simulink library "UserContent_lib"  (Simulink 7.2)
settings: Solver=ode45  SolverMode=SingleTasking  StartTime=0.0  StopTime=10.0  RelTol=1e-3
undefined symbols (not defined in the file or in its folder): bias, Timestep, WindDir, WindSpd
libraries: aeroutilslib x4, First_Order_Filter_lib x4, simulink x1, timer_lib x1
settings Model: Creator=Austin Murch  LastModifiedBy=la1032aw  ExtModeAutoUpdateStatusClock=off

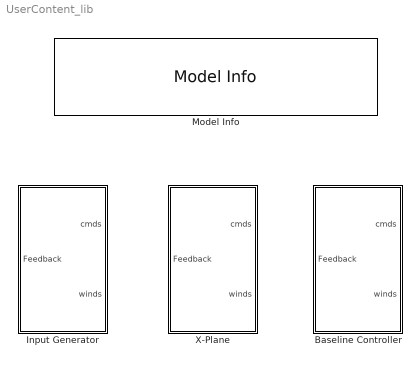
== system UserContent_lib ==
  Baseline Controller : Subsystem
  Input Generator : Subsystem
  Model Info : simulink/Model-Wide Utilities/Model Info  SystemSampleTime=-1  InitialBlockCM=None  BlockCM=None  Frame=on  DisplayStringWithTags=|  HorizontalTextAlignment=Center  LeftAlignmentValue=0.5  SourceBlockDiagram=UserContent_lib  TagMaxNumber=20
      | - gtm_design Input Library -
      | 
      | Model Version: %<ModelVersion>
      | Last modifed by %<LastModifiedBy> on %<LastModificationDate>
  X-Plane : Subsystem

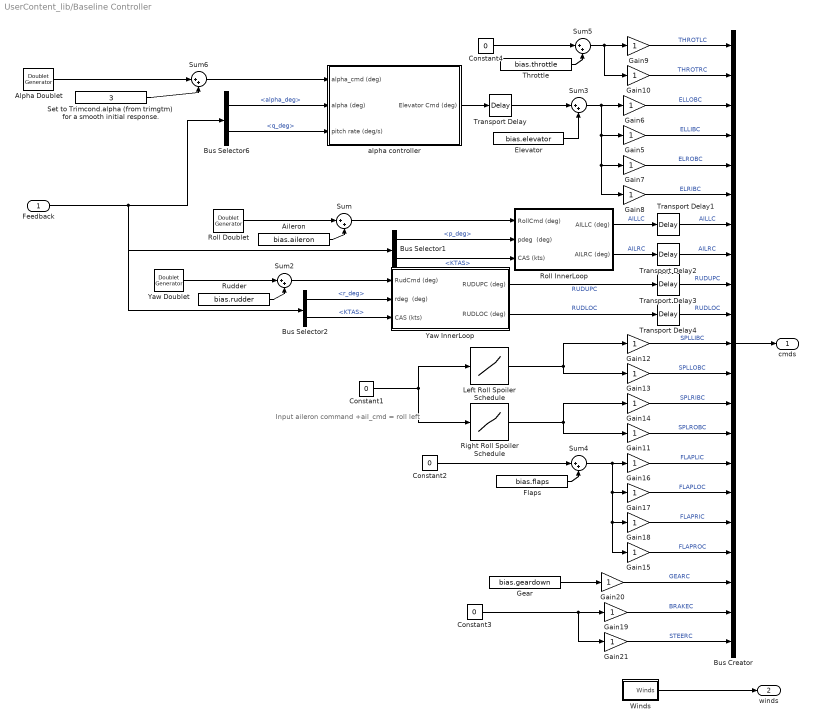
== system UserContent_lib/Baseline Controller ==
  note: Input aileron command
      | +ail_cmd = roll left
  Feedback : Inport  OutDataType=sfix(16)  OutScaling=2^0
  Aileron : Constant  Value=bias.aileron  OutDataType=sfix(16)  OutScaling=2^0
  Alpha Doublet : aeroutilslib/Doublet Generator  SystemSampleTime=-1  timeon=2  pulsewidth=2  amplitude=1
  Bus Creator : BusCreator  Inputs=21
  Bus Selector1 : BusSelector  OutputSignals=MAG3.p_deg,AirData.KTAS
  Bus Selector2 : BusSelector  OutputSignals=MAG3.r_deg,AirData.KTAS
  Bus Selector6 : BusSelector  OutputSignals=AirData.alpha_deg,MAG3.q_deg
  Constant{1..4} (4 alike) : Constant  Value=0  OutDataType=sfix(16)  OutScaling=2^0
  Elevator : Constant  Value=bias.elevator  OutDataType=sfix(16)  OutScaling=2^0
  Flaps : Constant  Value=bias.flaps  OutDataType=sfix(16)  OutScaling=2^0
  Gain{5..21} (17 alike) : Gain  ParameterDataType=sfix(16)  ParameterScaling=2^0  OutDataType=sfix(16)  OutScaling=2^0  SaturateOnIntegerOverflow=on  OutDataTypeStr=Inherit: Same as input  ParamDataTypeStr=Inherit: Same as input
  Gear : Constant  Value=bias.geardown  OutDataType=sfix(16)  OutScaling=2^0
  Left Roll Spoiler Schedule : Lookup  InputValues="[-20\t-11.76\t-2.36\t0\t2.36\t11.76\t20\t]"  Table=[0 0 0 0 0 9 45]  LookUpMeth=Interpolation-Use End Values  OutDataType=sfix(16)  OutScaling=2^0
  Right Roll Spoiler Schedule : Lookup  InputValues="[-20\t-11.76\t-2.36\t0\t2.36\t11.76\t20\t]"  Table=[45 9 0 0 0 0 0]  LookUpMeth=Interpolation-Use End Values  OutDataType=sfix(16)  OutScaling=2^0
  Roll Doublet : aeroutilslib/Doublet Generator  SystemSampleTime=-1  timeon=8  pulsewidth=2  amplitude=1
  Roll InnerLoop : Subsystem
  Rudder : Constant  Value=bias.rudder  OutDataType=sfix(16)  OutScaling=2^0
  Set to Trimcond.alpha (from trimgtm)  for a smooth initial response. : Constant  Value=3  OutDataType=sfix(16)  OutScaling=2^0
  Sum{,2..6} (6 alike) : Sum  Inputs=|++  OutDataType=sfix(16)  OutScaling=2^0
  Throttle : Constant  Value=bias.throttle  OutDataType=sfix(16)  OutScaling=2^0
  Transport Delay{,1..4} (5 alike) : TransportDelay  DelayTime=20e-3
  Winds : Subsystem
  Yaw Doublet : aeroutilslib/Doublet Generator  SystemSampleTime=-1  timeon=12  pulsewidth=2  amplitude=1
  Yaw InnerLoop : Subsystem
  alpha controller : Subsystem
  cmds : Outport  OutDataType=sfix(16)  OutScaling=2^0
  winds : Outport  Port=2  OutDataType=sfix(16)  OutScaling=2^0
  wires:
  Yaw Doublet/1 -> Sum2/1
  Roll Doublet/1 -> Sum/1
  Bus Selector2/2 -> Yaw InnerLoop/3(CAS (kts))  "<KTAS>"
  Bus Selector2/1 -> Yaw InnerLoop/2(rdeg  (deg))  "<r_deg>"
  Bus Selector1/2 -> Roll InnerLoop/3(CAS (kts))  "<KTAS>"
  Bus Selector1/1 -> Roll InnerLoop/2(pdeg  (deg))  "<p_deg>"
  Sum2/1 -> Yaw InnerLoop/1(RudCmd (deg))
  Rudder/1 -> Sum2/2
  Sum/1 -> Roll InnerLoop/1(RollCmd (deg))
  alpha controller/1(Elevator Cmd (deg)) -> Transport Delay/1
  Bus Selector6/1 -> alpha controller/2(alpha (deg))  "<alpha_deg>"
  Sum6/1 -> alpha controller/1(alpha_cmd (deg))
  Alpha Doublet/1 -> Sum6/1
  Set to Trimcond.alpha (from trimgtm)  for a smooth initial response./1 -> Sum6/2
  Gain12/1 -> Bus Creator/11  "SPLLIBC"
  Gain13/1 -> Bus Creator/12  "SPLLOBC"
  Gain14/1 -> Bus Creator/13  "SPLRIBC"
  Gain11/1 -> Bus Creator/14  "SPLROBC"
  Gain16/1 -> Bus Creator/15  "FLAPLIC"
  Gain17/1 -> Bus Creator/16  "FLAPLOC"
  Gain18/1 -> Bus Creator/17  "FLAPRIC"
  Gain15/1 -> Bus Creator/18  "FLAPROC"
  Gain9/1 -> Bus Creator/1  "THROTLC"
  Gain10/1 -> Bus Creator/2  "THROTRC"
  Gain5/1 -> Bus Creator/4  "ELLIBC"
  Gain6/1 -> Bus Creator/3  "ELLOBC"
  Gain7/1 -> Bus Creator/5  "ELROBC"
  Gain8/1 -> Bus Creator/6  "ELRIBC"
  Roll InnerLoop/1(AILLC (deg)) -> Transport Delay1/1  "AILLC"
  Roll InnerLoop/2(AILRC (deg)) -> Transport Delay2/1  "AILRC"
  Yaw InnerLoop/1(RUDUPC (deg)) -> Transport Delay3/1  "RUDUPC"
  Yaw InnerLoop/2(RUDLOC (deg)) -> Transport Delay4/1  "RUDLOC"
  Throttle/1 -> Sum5/2
  Constant4/1 -> Sum5/1
  Sum5/1 -> Gain10/1, Gain9/1
  Sum3/1 -> Gain6/1, Gain5/1, Gain7/1, Gain8/1
  Aileron/1 -> Sum/2
  Elevator/1 -> Sum3/2
  Flaps/1 -> Sum4/2
  Constant2/1 -> Sum4/1
  Sum4/1 -> Gain16/1, Gain17/1, Gain18/1, Gain15/1
  Gain19/1 -> Bus Creator/20  "BRAKEC"
  Gear/1 -> Gain20/1
  Constant3/1 -> Gain19/1, Gain21/1
  Bus Creator/1 -> cmds/1
  Feedback/1 -> Bus Selector6/1, Bus Selector2/1, Bus Selector1/1
  Gain20/1 -> Bus Creator/19  "GEARC"
  Gain21/1 -> Bus Creator/21  "STEERC"
  Bus Selector6/2 -> alpha controller/3(pitch rate (deg/s))  "<q_deg>"
  Left Roll Spoiler Schedule/1 -> Gain12/1, Gain13/1
  Right Roll Spoiler Schedule/1 -> Gain14/1, Gain11/1
  Constant1/1 -> Left Roll Spoiler Schedule/1, Right Roll Spoiler Schedule/1
  Winds/1(Winds) -> winds/1
  Transport Delay/1 -> Sum3/1
  Transport Delay1/1 -> Bus Creator/7  "AILLC"
  Transport Delay2/1 -> Bus Creator/8  "AILRC"
  Transport Delay4/1 -> Bus Creator/10  "RUDLOC"
  Transport Delay3/1 -> Bus Creator/9  "RUDUPC"

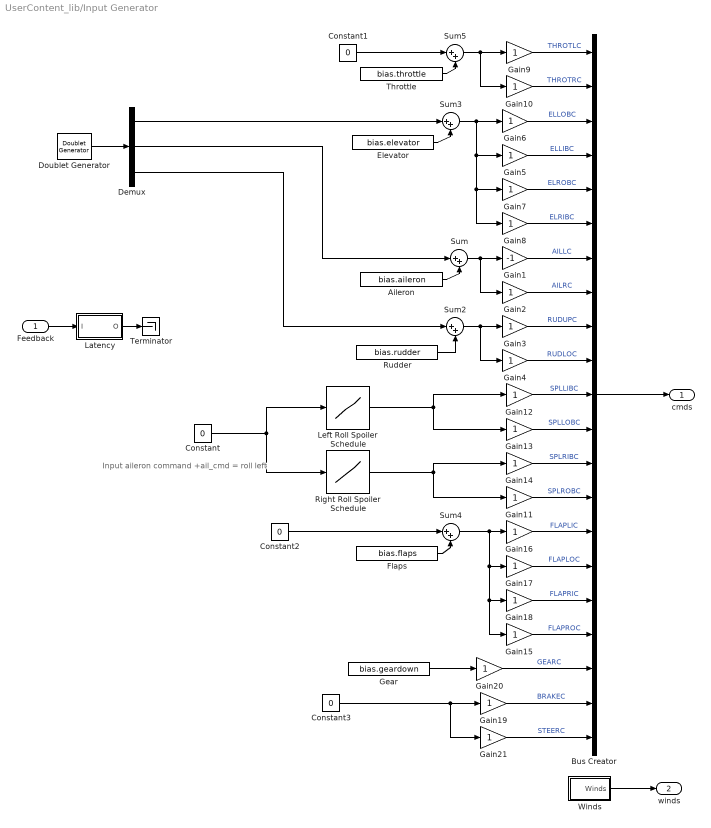
== system UserContent_lib/Input Generator ==
  note: Input aileron command
      | +ail_cmd = roll left
  Feedback : Inport  OutDataType=sfix(16)  OutScaling=2^0
  Aileron : Constant  Value=bias.aileron  OutDataType=sfix(16)  OutScaling=2^0
  Bus Creator : BusCreator  Inputs=21
  Constant{,1..3} (4 alike) : Constant  Value=0  OutDataType=sfix(16)  OutScaling=2^0
  Demux : Demux  Outputs=3
  Doublet Generator : aeroutilslib/Doublet Generator  SystemSampleTime=-1  timeon=[2 10 18]  pulsewidth=[2 2 2]  amplitude=[0 0 0]
  Elevator : Constant  Value=bias.elevator  OutDataType=sfix(16)  OutScaling=2^0
  Flaps : Constant  Value=bias.flaps  OutDataType=sfix(16)  OutScaling=2^0
  Gain1 : Gain  Gain=-1  ParameterDataType=sfix(16)  ParameterScaling=2^0  OutDataType=sfix(16)  OutScaling=2^0  SaturateOnIntegerOverflow=on  OutDataTypeStr=Inherit: Same as input  ParamDataTypeStr=Inherit: Same as input
  Gain{2..21} (20 alike) : Gain  ParameterDataType=sfix(16)  ParameterScaling=2^0  OutDataType=sfix(16)  OutScaling=2^0  SaturateOnIntegerOverflow=on  OutDataTypeStr=Inherit: Same as input  ParamDataTypeStr=Inherit: Same as input
  Gear : Constant  Value=bias.geardown  OutDataType=sfix(16)  OutScaling=2^0
  Latency : Subsystem
  Left Roll Spoiler Schedule : Lookup  InputValues="[-20\t-11.76\t-2.36\t0\t2.36\t11.76\t20\t]"  Table=[0 0 0 0 0 9 45]  LookUpMeth=Interpolation-Use End Values  OutDataType=sfix(16)  OutScaling=2^0
  Right Roll Spoiler Schedule : Lookup  InputValues="[-20\t-11.76\t-2.36\t0\t2.36\t11.76\t20\t]"  Table=[45 9 0 0 0 0 0]  LookUpMeth=Interpolation-Use End Values  OutDataType=sfix(16)  OutScaling=2^0
  Rudder : Constant  Value=bias.rudder  OutDataType=sfix(16)  OutScaling=2^0
  Sum{,2..5} (5 alike) : Sum  Inputs=|++  OutDataType=sfix(16)  OutScaling=2^0
  Terminator : Terminator
  Throttle : Constant  Value=bias.throttle  OutDataType=sfix(16)  OutScaling=2^0
  Winds : Subsystem
  cmds : Outport  OutDataType=sfix(16)  OutScaling=2^0
  winds : Outport  Port=2  OutDataType=sfix(16)  OutScaling=2^0
  wires:
  Gain21/1 -> Bus Creator/21  "STEERC"
  Gain20/1 -> Bus Creator/19  "GEARC"
  Feedback/1 -> Latency/1(I)
  Bus Creator/1 -> cmds/1
  Demux/1 -> Sum3/1
  Constant3/1 -> Gain21/1, Gain19/1
  Gear/1 -> Gain20/1
  Gain19/1 -> Bus Creator/20  "BRAKEC"
  Demux/3 -> Sum2/1
  Demux/2 -> Sum/1
  Doublet Generator/1 -> Demux/1
  Sum4/1 -> Gain15/1, Gain18/1, Gain17/1, Gain16/1
  Constant2/1 -> Sum4/1
  Flaps/1 -> Sum4/2
  Rudder/1 -> Sum2/2
  Sum2/1 -> Gain4/1, Gain3/1
  Sum/1 -> Gain2/1, Gain1/1
  Elevator/1 -> Sum3/2
  Aileron/1 -> Sum/2
  Sum3/1 -> Gain8/1, Gain7/1, Gain5/1, Gain6/1
  Sum5/1 -> Gain9/1, Gain10/1
  Constant1/1 -> Sum5/1
  Throttle/1 -> Sum5/2
  Gain4/1 -> Bus Creator/10  "RUDLOC"
  Gain3/1 -> Bus Creator/9  "RUDUPC"
  Gain2/1 -> Bus Creator/8  "AILRC"
  Gain1/1 -> Bus Creator/7  "AILLC"
  Gain8/1 -> Bus Creator/6  "ELRIBC"
  Gain7/1 -> Bus Creator/5  "ELROBC"
  Gain6/1 -> Bus Creator/3  "ELLOBC"
  Gain5/1 -> Bus Creator/4  "ELLIBC"
  Gain10/1 -> Bus Creator/2  "THROTRC"
  Gain9/1 -> Bus Creator/1  "THROTLC"
  Gain15/1 -> Bus Creator/18  "FLAPROC"
  Gain18/1 -> Bus Creator/17  "FLAPRIC"
  Gain17/1 -> Bus Creator/16  "FLAPLOC"
  Gain16/1 -> Bus Creator/15  "FLAPLIC"
  Gain11/1 -> Bus Creator/14  "SPLROBC"
  Gain14/1 -> Bus Creator/13  "SPLRIBC"
  Gain13/1 -> Bus Creator/12  "SPLLOBC"
  Gain12/1 -> Bus Creator/11  "SPLLIBC"
  Left Roll Spoiler Schedule/1 -> Gain12/1, Gain13/1
  Right Roll Spoiler Schedule/1 -> Gain14/1, Gain11/1
  Constant/1 -> Left Roll Spoiler Schedule/1, Right Roll Spoiler Schedule/1
  Winds/1(Winds) -> winds/1
  Latency/1(O) -> Terminator/1

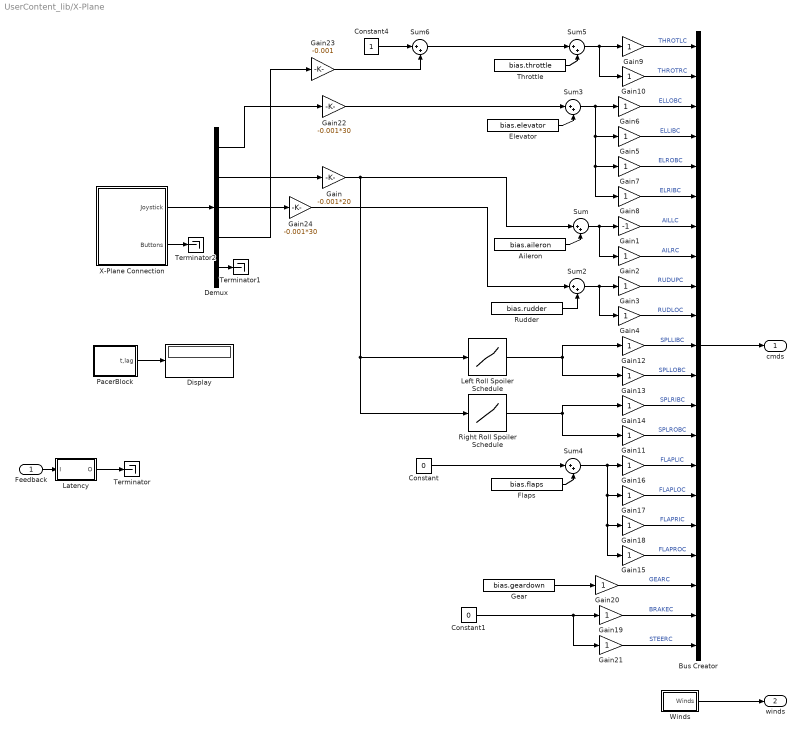
== system UserContent_lib/X-Plane ==
  Feedback : Inport  OutDataType=sfix(16)  OutScaling=2^0
  Aileron : Constant  Value=bias.aileron  OutDataType=sfix(16)  OutScaling=2^0
  Bus Creator : BusCreator  Inputs=21
  Constant : Constant  Value=0  OutDataType=sfix(16)  OutScaling=2^0
  Constant1 : Constant  Value=0  OutDataType=sfix(16)  OutScaling=2^0
  Constant4 : Constant  OutDataType=sfix(16)  OutScaling=2^0
  Demux : Demux  Outputs=[1 1 1 1 -1]
  Display : Display
  Elevator : Constant  Value=bias.elevator  OutDataType=sfix(16)  OutScaling=2^0
  Flaps : Constant  Value=bias.flaps  OutDataType=sfix(16)  OutScaling=2^0
  Gain : Gain  Gain=-0.001*20  ParameterDataType=sfix(16)  ParameterScaling=2^0  OutDataType=sfix(16)  OutScaling=2^0
  Gain1 : Gain  Gain=-1  ParameterDataType=sfix(16)  ParameterScaling=2^0  OutDataType=sfix(16)  OutScaling=2^0  SaturateOnIntegerOverflow=on  OutDataTypeStr=Inherit: Same as input  ParamDataTypeStr=Inherit: Same as input
  Gain{2..21} (20 alike) : Gain  ParameterDataType=sfix(16)  ParameterScaling=2^0  OutDataType=sfix(16)  OutScaling=2^0  SaturateOnIntegerOverflow=on  OutDataTypeStr=Inherit: Same as input  ParamDataTypeStr=Inherit: Same as input
  Gain22 : Gain  Gain=-0.001*30  ParameterDataType=sfix(16)  ParameterScaling=2^0  OutDataType=sfix(16)  OutScaling=2^0
  Gain23 : Gain  Gain=-0.001  ParameterDataType=sfix(16)  ParameterScaling=2^0  OutDataType=sfix(16)  OutScaling=2^0
  Gain24 : Gain  Gain=-0.001*30  ParameterDataType=sfix(16)  ParameterScaling=2^0  OutDataType=sfix(16)  OutScaling=2^0
  Gear : Constant  Value=bias.geardown  OutDataType=sfix(16)  OutScaling=2^0
  Latency : Subsystem
  Left Roll Spoiler Schedule : Lookup  InputValues="[-20\t-11.76\t-2.36\t0\t2.36\t11.76\t20\t]"  Table=[0 0 0 0 0 9 45]  LookUpMeth=Interpolation-Use End Values  OutDataType=sfix(16)  OutScaling=2^0
  PacerBlock : Subsystem  BlockChoice=RealTimeSpeed
      settings: AttributesFormatString=%<BlockChoice>  TemplateBlock=timer_lib/PacerBlock  MemberBlocks=RealTimeSpeed,SimTimeSpeed
  Right Roll Spoiler Schedule : Lookup  InputValues="[-20\t-11.76\t-2.36\t0\t2.36\t11.76\t20\t]"  Table=[45 9 0 0 0 0 0]  LookUpMeth=Interpolation-Use End Values  OutDataType=sfix(16)  OutScaling=2^0
  Rudder : Constant  Value=bias.rudder  OutDataType=sfix(16)  OutScaling=2^0
  Sum{,2..6} (6 alike) : Sum  Inputs=|++  OutDataType=sfix(16)  OutScaling=2^0
  Terminator : Terminator
  Terminator1 : Terminator
  Terminator2 : Terminator
  Throttle : Constant  Value=bias.throttle  OutDataType=sfix(16)  OutScaling=2^0
  Winds : Subsystem
  X-Plane Connection : Subsystem
  cmds : Outport  OutDataType=sfix(16)  OutScaling=2^0
  winds : Outport  Port=2  OutDataType=sfix(16)  OutScaling=2^0
  wires:
  Latency/1(O) -> Terminator/1
  PacerBlock/1(t,lag) -> Display/1
  X-Plane Connection/2(Buttons) -> Terminator2/1
  X-Plane Connection/1(Joystick) -> Demux/1
  Gain23/1 -> Sum6/2
  Constant4/1 -> Sum6/1
  Sum6/1 -> Sum5/1
  Gain24/1 -> Sum2/1
  Gain22/1 -> Sum3/1
  Gain/1 -> Sum/1, Left Roll Spoiler Schedule/1, Right Roll Spoiler Schedule/1
  Demux/2 -> Gain/1
  Demux/1 -> Gain22/1
  Demux/5 -> Terminator1/1
  Demux/4 -> Gain23/1
  Demux/3 -> Gain24/1
  Gain12/1 -> Bus Creator/11  "SPLLIBC"
  Gain13/1 -> Bus Creator/12  "SPLLOBC"
  Gain14/1 -> Bus Creator/13  "SPLRIBC"
  Gain11/1 -> Bus Creator/14  "SPLROBC"
  Gain16/1 -> Bus Creator/15  "FLAPLIC"
  Gain17/1 -> Bus Creator/16  "FLAPLOC"
  Gain18/1 -> Bus Creator/17  "FLAPRIC"
  Gain15/1 -> Bus Creator/18  "FLAPROC"
  Gain9/1 -> Bus Creator/1  "THROTLC"
  Gain10/1 -> Bus Creator/2  "THROTRC"
  Gain5/1 -> Bus Creator/4  "ELLIBC"
  Gain6/1 -> Bus Creator/3  "ELLOBC"
  Gain7/1 -> Bus Creator/5  "ELROBC"
  Gain8/1 -> Bus Creator/6  "ELRIBC"
  Gain1/1 -> Bus Creator/7  "AILLC"
  Gain2/1 -> Bus Creator/8  "AILRC"
  Gain3/1 -> Bus Creator/9  "RUDUPC"
  Gain4/1 -> Bus Creator/10  "RUDLOC"
  Throttle/1 -> Sum5/2
  Sum5/1 -> Gain10/1, Gain9/1
  Sum3/1 -> Gain6/1, Gain5/1, Gain7/1, Gain8/1
  Aileron/1 -> Sum/2
  Elevator/1 -> Sum3/2
  Sum/1 -> Gain1/1, Gain2/1
  Sum2/1 -> Gain3/1, Gain4/1
  Rudder/1 -> Sum2/2
  Flaps/1 -> Sum4/2
  Constant/1 -> Sum4/1
  Sum4/1 -> Gain16/1, Gain17/1, Gain18/1, Gain15/1
  Gain19/1 -> Bus Creator/20  "BRAKEC"
  Gear/1 -> Gain20/1
  Constant1/1 -> Gain19/1, Gain21/1
  Bus Creator/1 -> cmds/1
  Feedback/1 -> Latency/1(I)
  Gain20/1 -> Bus Creator/19  "GEARC"
  Gain21/1 -> Bus Creator/21  "STEERC"
  Left Roll Spoiler Schedule/1 -> Gain12/1, Gain13/1
  Right Roll Spoiler Schedule/1 -> Gain14/1, Gain11/1
  Winds/1(Winds) -> winds/1

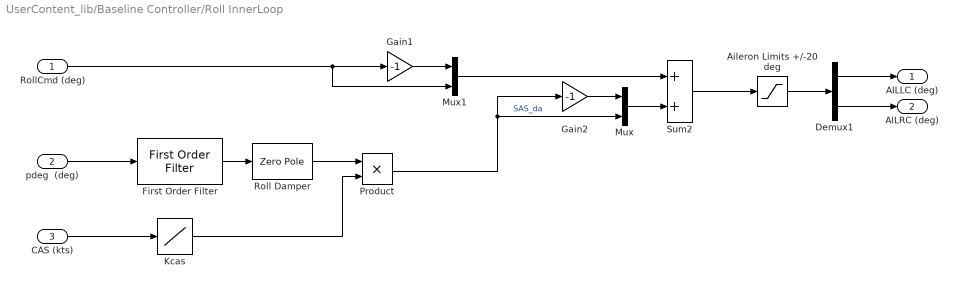
== system UserContent_lib/Baseline Controller/Roll InnerLoop ==
  RollCmd (deg) : Inport  OutDataType=sfix(16)  OutScaling=2^0
  pdeg  (deg) : Inport  Port=2  OutDataType=sfix(16)  OutScaling=2^0
  CAS (kts) : Inport  Port=3  OutDataType=sfix(16)  OutScaling=2^0
  Aileron Limits +/-20 deg : Saturate  UpperLimit=20  LowerLimit=-20
  Demux1 : Demux  Outputs=2
  First Order Filter : First_Order_Filter_lib/First Order Filter  SystemSampleTime=-1  tau=1/(4*pi)  timestep=Timestep
  Gain1 : Gain  Gain=-1  ParameterDataType=sfix(16)  ParameterScaling=2^0  OutDataType=sfix(16)  OutScaling=2^0
  Gain2 : Gain  Gain=-1  ParameterDataType=sfix(16)  ParameterScaling=2^0  OutDataType=sfix(16)  OutScaling=2^0
  Kcas : Lookup  InputValues=[0 50 100]  Table=[1.0 1.0 0]  LookUpMeth=Interpolation-Use End Values  OutDataType=sfix(16)  OutScaling=2^0
  Mux : Mux  Inputs=2
  Mux1 : Mux  Inputs=2
  Product : Product  OutDataType=sfix(16)  OutScaling=2^0  RndMeth=Zero
  Roll Damper : ZeroPole  Zeros=0  Poles=-5  Gain=0.1
  Sum2 : Sum  OutDataType=sfix(16)  OutScaling=2^0
  AILLC (deg) : Outport  OutDataType=sfix(16)  OutScaling=2^0
  AILRC (deg) : Outport  Port=2  OutDataType=sfix(16)  OutScaling=2^0
  wires:
  Sum2/1 -> Aileron Limits +/-20 deg/1
  Mux/1 -> Sum2/2
  Gain2/1 -> Mux/1
  Demux1/2 -> AILRC (deg)/1
  Aileron Limits +/-20 deg/1 -> Demux1/1
  Demux1/1 -> AILLC (deg)/1
  First Order Filter/1 -> Roll Damper/1
  Roll Damper/1 -> Product/1
  Kcas/1 -> Product/2
  CAS (kts)/1 -> Kcas/1
  pdeg  (deg)/1 -> First Order Filter/1
  Product/1 -> Mux/2, Gain2/1  "SAS_da"
  Mux1/1 -> Sum2/1
  Gain1/1 -> Mux1/1
  RollCmd (deg)/1 -> Gain1/1, Mux1/2

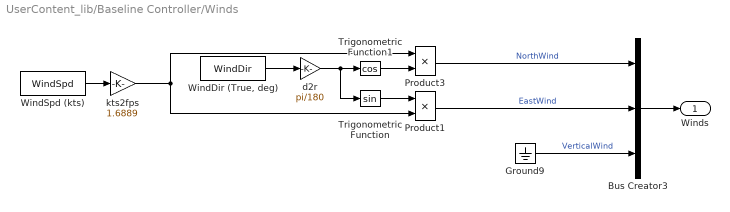
== system UserContent_lib/Baseline Controller/Winds ==
  Bus Creator3 : BusCreator  Inputs=3
  Ground9 : Ground
  Product1 : Product  Inputs=**  OutDataType=sfix(16)  OutScaling=2^0  SaturateOnIntegerOverflow=on  InputSameDT=on  OutDataTypeStr=Inherit: Same as first input
  Product3 : Product  Inputs=**  OutDataType=sfix(16)  OutScaling=2^0  SaturateOnIntegerOverflow=on  InputSameDT=on  OutDataTypeStr=Inherit: Same as first input
  Trigonometric Function : Trigonometry
  Trigonometric Function1 : Trigonometry  Operator=cos
  "WindDir (True, deg)" : Constant  Value=WindDir  OutDataType=sfix(16)  OutScaling=2^0
  WindSpd (kts) : Constant  Value=WindSpd  OutDataType=sfix(16)  OutScaling=2^0
  d2r : Gain  Gain=pi/180  ParameterDataType=sfix(16)  ParameterScaling=2^0  OutDataType=sfix(16)  OutScaling=2^0  SaturateOnIntegerOverflow=on  OutDataTypeStr=Inherit: Same as input  ParamDataTypeStr=Inherit: Same as input
  kts2fps : Gain  Gain=1.6889  ParameterDataType=sfix(16)  ParameterScaling=2^0  OutDataType=sfix(16)  OutScaling=2^0  SaturateOnIntegerOverflow=on  OutDataTypeStr=Inherit: Same as input  ParamDataTypeStr=Inherit: Same as input
  Winds : Outport  OutDataType=sfix(16)  OutScaling=2^0
  wires:
  kts2fps/1 -> Product1/2, Product3/1
  WindSpd (kts)/1 -> kts2fps/1
  "WindDir (True, deg)"/1 -> d2r/1
  d2r/1 -> Trigonometric Function1/1, Trigonometric Function/1
  Trigonometric Function1/1 -> Product3/2
  Trigonometric Function/1 -> Product1/1
  Bus Creator3/1 -> Winds/1
  Ground9/1 -> Bus Creator3/3  "VerticalWind"
  Product1/1 -> Bus Creator3/2  "EastWind"
  Product3/1 -> Bus Creator3/1  "NorthWind"

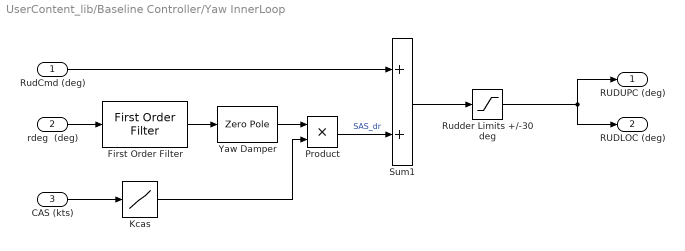
== system UserContent_lib/Baseline Controller/Yaw InnerLoop ==
  RudCmd (deg) : Inport  OutDataType=sfix(16)  OutScaling=2^0
  rdeg  (deg) : Inport  Port=2  OutDataType=sfix(16)  OutScaling=2^0
  CAS (kts) : Inport  Port=3  OutDataType=sfix(16)  OutScaling=2^0
  First Order Filter : First_Order_Filter_lib/First Order Filter  SystemSampleTime=-1  tau=1/(4*pi)  timestep=Timestep
  Kcas : Lookup  InputValues=[0 60 120]  Table=[1.0 1.0 0]  LookUpMeth=Interpolation-Use End Values  OutDataType=sfix(16)  OutScaling=2^0
  Product : Product  OutDataType=sfix(16)  OutScaling=2^0  RndMeth=Zero
  Rudder Limits +/-30 deg : Saturate  UpperLimit=30  LowerLimit=-30
  Sum1 : Sum  OutDataType=sfix(16)  OutScaling=2^0
  Yaw Damper : ZeroPole  Zeros=0  Poles=-5  Gain=0.2
  RUDUPC (deg) : Outport  OutDataType=sfix(16)  OutScaling=2^0
  RUDLOC (deg) : Outport  Port=2  OutDataType=sfix(16)  OutScaling=2^0
  wires:
  Rudder Limits +/-30 deg/1 -> RUDUPC (deg)/1, RUDLOC (deg)/1
  RudCmd (deg)/1 -> Sum1/1
  Product/1 -> Sum1/2  "SAS_dr"
  First Order Filter/1 -> Yaw Damper/1
  Yaw Damper/1 -> Product/1
  Kcas/1 -> Product/2
  Sum1/1 -> Rudder Limits +/-30 deg/1
  CAS (kts)/1 -> Kcas/1
  rdeg  (deg)/1 -> First Order Filter/1

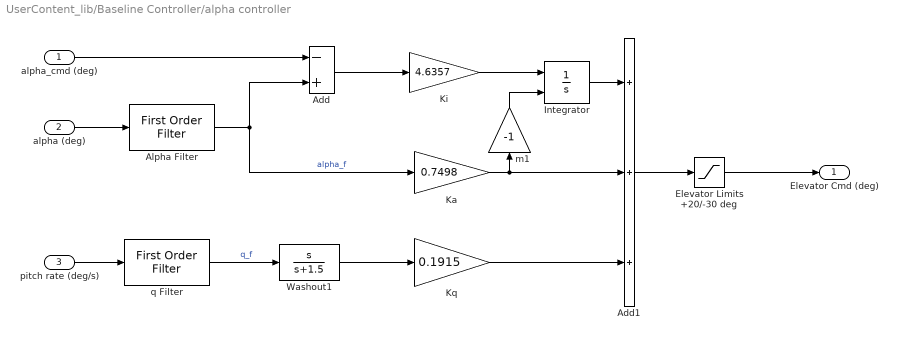
== system UserContent_lib/Baseline Controller/alpha controller ==
  alpha_cmd (deg) : Inport  OutDataType=sfix(16)  OutScaling=2^0
  alpha (deg) : Inport  Port=2  OutDataType=sfix(16)  OutScaling=2^0
  pitch rate (deg/s) : Inport  Port=3  OutDataType=sfix(16)  OutScaling=2^0
  " q Filter" : First_Order_Filter_lib/First Order Filter  SystemSampleTime=-1  tau=1/(8*pi)  timestep=Timestep
  Add : Sum  Inputs=-+  OutDataType=sfix(16)  OutScaling=2^-10
  Add1 : Sum  Inputs=+++  OutDataType=sfix(16)  OutScaling=2^-10
  Alpha Filter : First_Order_Filter_lib/First Order Filter  SystemSampleTime=-1  tau=1/(8*pi)  timestep=Timestep
  Elevator Limits +20/-30 deg : Saturate  UpperLimit=20  LowerLimit=-30
  Integrator : Integrator  InitialConditionSource=external  InitialCondition=-0.7498*4.64
  Ka : Gain  Gain=0.7498  ParameterDataType=sfix(16)  ParameterScaling=2^0  OutDataType=sfix(16)  OutScaling=2^0
  Ki : Gain  Gain=4.6357  ParameterDataType=sfix(16)  ParameterScaling=2^0  OutDataType=sfix(16)  OutScaling=2^0
  Kq : Gain  Gain=0.1915  ParameterDataType=sfix(16)  ParameterScaling=2^0  OutDataType=sfix(16)  OutScaling=2^0
  Washout1 : TransferFcn  Numerator=[1 0]  Denominator=[1 1.5]
  m1 : Gain  Orientation=up  Gain=-1  ParameterDataType=sfix(16)  ParameterScaling=2^0  OutDataType=sfix(16)  OutScaling=2^0
  Elevator Cmd (deg) : Outport  OutDataType=sfix(16)  OutScaling=2^0
  wires:
  m1/1 -> Integrator/2
  Elevator Limits +20/-30 deg/1 -> Elevator Cmd (deg)/1
  Washout1/1 -> Kq/1
  pitch rate (deg/s)/1 -> " q Filter"/1
  Alpha Filter/1 -> Ka/1, Add/2  "alpha_f"
  " q Filter"/1 -> Washout1/1  "q_f"
  Add1/1 -> Elevator Limits +20/-30 deg/1
  Kq/1 -> Add1/3
  Ka/1 -> m1/1, Add1/2
  Integrator/1 -> Add1/1
  Ki/1 -> Integrator/1
  Add/1 -> Ki/1
  alpha_cmd (deg)/1 -> Add/1
  alpha (deg)/1 -> Alpha Filter/1

== system UserContent_lib/Input Generator/Latency ==
  I : Inport  OutDataType=sfix(16)  OutScaling=2^0
  Unit Delay{,1..3} (4 alike) : UnitDelay  SampleTime=Timestep
  O : Outport  OutDataType=sfix(16)  OutScaling=2^0
  wires:
  I/1 -> Unit Delay/1
  Unit Delay/1 -> Unit Delay1/1
  Unit Delay1/1 -> Unit Delay2/1
  Unit Delay2/1 -> Unit Delay3/1
  Unit Delay3/1 -> O/1

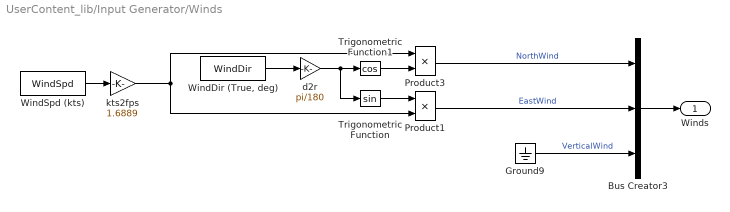
== system UserContent_lib/Input Generator/Winds ==
  Bus Creator3 : BusCreator  Inputs=3
  Ground9 : Ground
  Product1 : Product  Inputs=**  OutDataType=sfix(16)  OutScaling=2^0  SaturateOnIntegerOverflow=on  InputSameDT=on  OutDataTypeStr=Inherit: Same as first input
  Product3 : Product  Inputs=**  OutDataType=sfix(16)  OutScaling=2^0  SaturateOnIntegerOverflow=on  InputSameDT=on  OutDataTypeStr=Inherit: Same as first input
  Trigonometric Function : Trigonometry
  Trigonometric Function1 : Trigonometry  Operator=cos
  "WindDir (True, deg)" : Constant  Value=WindDir  OutDataType=sfix(16)  OutScaling=2^0
  WindSpd (kts) : Constant  Value=WindSpd  OutDataType=sfix(16)  OutScaling=2^0
  d2r : Gain  Gain=pi/180  ParameterDataType=sfix(16)  ParameterScaling=2^0  OutDataType=sfix(16)  OutScaling=2^0  SaturateOnIntegerOverflow=on  OutDataTypeStr=Inherit: Same as input  ParamDataTypeStr=Inherit: Same as input
  kts2fps : Gain  Gain=1.6889  ParameterDataType=sfix(16)  ParameterScaling=2^0  OutDataType=sfix(16)  OutScaling=2^0  SaturateOnIntegerOverflow=on  OutDataTypeStr=Inherit: Same as input  ParamDataTypeStr=Inherit: Same as input
  Winds : Outport  OutDataType=sfix(16)  OutScaling=2^0
  wires:
  Product3/1 -> Bus Creator3/1  "NorthWind"
  Product1/1 -> Bus Creator3/2  "EastWind"
  Ground9/1 -> Bus Creator3/3  "VerticalWind"
  Bus Creator3/1 -> Winds/1
  Trigonometric Function/1 -> Product1/1
  Trigonometric Function1/1 -> Product3/2
  d2r/1 -> Trigonometric Function/1, Trigonometric Function1/1
  "WindDir (True, deg)"/1 -> d2r/1
  WindSpd (kts)/1 -> kts2fps/1
  kts2fps/1 -> Product3/1, Product1/2

== system UserContent_lib/X-Plane/Latency ==
  I : Inport  OutDataType=sfix(16)  OutScaling=2^0
  Unit Delay{,1..3} (4 alike) : UnitDelay  SampleTime=Timestep
  O : Outport  OutDataType=sfix(16)  OutScaling=2^0
  wires:
  I/1 -> Unit Delay/1
  Unit Delay/1 -> Unit Delay1/1
  Unit Delay1/1 -> Unit Delay2/1
  Unit Delay2/1 -> Unit Delay3/1
  Unit Delay3/1 -> O/1

== system UserContent_lib/X-Plane/PacerBlock ==
  RealTimeSpeed : timer_lib/RealTimeSpeed  SystemSampleTime=-1
  t,lag : Outport  OutDataType=sfix(16)  OutScaling=2^0
  wires:
  RealTimeSpeed/1 -> t,lag/1

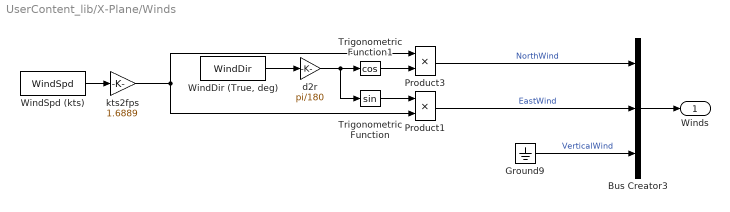
== system UserContent_lib/X-Plane/Winds ==
  Bus Creator3 : BusCreator  Inputs=3
  Ground9 : Ground
  Product1 : Product  Inputs=**  OutDataType=sfix(16)  OutScaling=2^0  SaturateOnIntegerOverflow=on  InputSameDT=on  OutDataTypeStr=Inherit: Same as first input
  Product3 : Product  Inputs=**  OutDataType=sfix(16)  OutScaling=2^0  SaturateOnIntegerOverflow=on  InputSameDT=on  OutDataTypeStr=Inherit: Same as first input
  Trigonometric Function : Trigonometry
  Trigonometric Function1 : Trigonometry  Operator=cos
  "WindDir (True, deg)" : Constant  Value=WindDir  OutDataType=sfix(16)  OutScaling=2^0
  WindSpd (kts) : Constant  Value=WindSpd  OutDataType=sfix(16)  OutScaling=2^0
  d2r : Gain  Gain=pi/180  ParameterDataType=sfix(16)  ParameterScaling=2^0  OutDataType=sfix(16)  OutScaling=2^0  SaturateOnIntegerOverflow=on  OutDataTypeStr=Inherit: Same as input  ParamDataTypeStr=Inherit: Same as input
  kts2fps : Gain  Gain=1.6889  ParameterDataType=sfix(16)  ParameterScaling=2^0  OutDataType=sfix(16)  OutScaling=2^0  SaturateOnIntegerOverflow=on  OutDataTypeStr=Inherit: Same as input  ParamDataTypeStr=Inherit: Same as input
  Winds : Outport  OutDataType=sfix(16)  OutScaling=2^0
  wires:
  kts2fps/1 -> Product1/2, Product3/1
  WindSpd (kts)/1 -> kts2fps/1
  "WindDir (True, deg)"/1 -> d2r/1
  d2r/1 -> Trigonometric Function1/1, Trigonometric Function/1
  Trigonometric Function1/1 -> Product3/2
  Trigonometric Function/1 -> Product1/1
  Bus Creator3/1 -> Winds/1
  Ground9/1 -> Bus Creator3/3  "VerticalWind"
  Product1/1 -> Bus Creator3/2  "EastWind"
  Product3/1 -> Bus Creator3/1  "NorthWind"

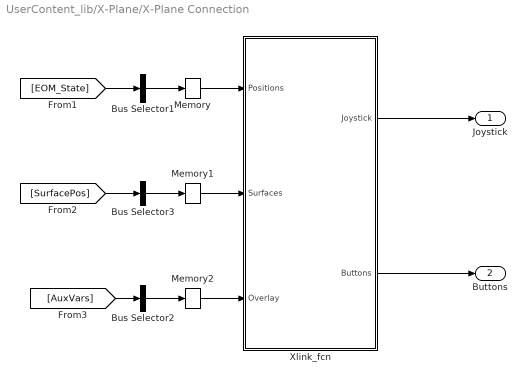
== system UserContent_lib/X-Plane/X-Plane Connection ==
  Bus Selector1 : BusSelector  OutputSignals=latitude,longitude,altitude,phi,theta,psi  OutputAsBus=on
  Bus Selector2 : BusSelector  OutputSignals=alpha,beta,tas  OutputAsBus=on
  Bus Selector3 : BusSelector  OutputSignals=AILL,ELLOB,RUDU,FLAPLIB,SPLLIB,GEAR  OutputAsBus=on
  Memory : Memory
  Memory1 : Memory
  Memory2 : Memory
  Xlink_fcn : Subsystem  mask(Xlink){HUDCell={'alpha','beta','Velocity'}}
      mask prompts: HUDCell "Lables for HUD, (cell array)"
      mask help:
      | Input Positions and Surfaces for X-Plane Visualization.
      |   Positions - [ Latitude, Longitude, Altitude, Roll, Pitch, Yaw] % degrees and ft.
      |   Surfaces  - [ Aileron, Elevator, Rudder, Flaps, Spoiler, GearDown] % deg and 0/1
      |
      | Output is Joysick axes and Button pushes.
      |   Joystick - First 16 axes
      |   Buttons  - 16 buttons as assigned to Xlink in X-Plane
      mask init:
      | if isempty(HUDCell) HUDCell=cell(6,1); end
      | HUDTextArray = uint8(zeros(90,1));
      | 
      | % loop through names, assign to string arrays
      | for i=1:min(length(HUDCell),6);
      |   if length(HUDCell{i})>14 HUDCell{i}=HUDCell{i}(1:14); end
      |   if length(HUDCell{i}>0),
      |     HUDTextArray((i-1)*15+1:(i-1)*15+length(HUDCell{i})) = uint8(HUDCell{i});
      |   end
      | end
  Joystick : Outport  OutDataType=sfix(16)  OutScaling=2^0
  Buttons : Outport  Port=2  OutDataType=sfix(16)  OutScaling=2^0
  wires:
  Memory2/1 -> Xlink_fcn/3(Overlay)
  Memory1/1 -> Xlink_fcn/2(Surfaces)
  Memory/1 -> Xlink_fcn/1(Positions)
  [AuxVars] -> Bus Selector2/1
  Bus Selector3/1 -> Memory1/1
  [EOM_State] -> Bus Selector1/1
  [SurfacePos] -> Bus Selector3/1
  Bus Selector2/1 -> Memory2/1
  Bus Selector1/1 -> Memory/1
  Xlink_fcn/2(Buttons) -> Buttons/1
  Xlink_fcn/1(Joystick) -> Joystick/1

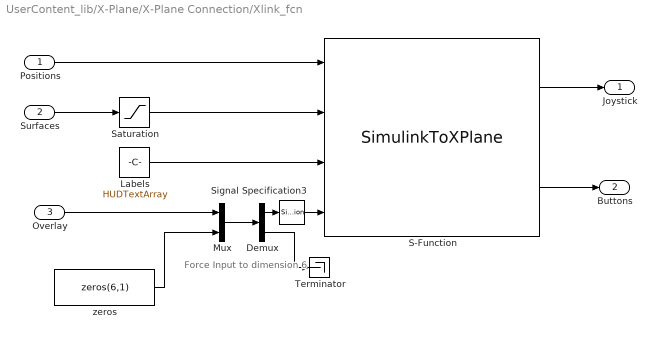
== system UserContent_lib/X-Plane/X-Plane Connection/Xlink_fcn ==
  note: Force Input to
      | dimension 6
  Positions : Inport  OutDataType=sfix(16)  OutScaling=2^0
  Surfaces : Inport  Port=2  OutDataType=sfix(16)  OutScaling=2^0
  Overlay : Inport  Port=3  OutDataType=sfix(16)  OutScaling=2^0
  Demux : Demux  Outputs=[6 -1]
  Labels : Constant  Value=HUDTextArray  OutDataTypeMode=uint8  OutDataType=sfix(16)  OutScaling=2^0  OutDataTypeStr=uint8
  Mux : Mux  Inputs=2
  S-Function : S-Function  FunctionName=SimulinkToXPlane  EnableBusSupport=off
  Saturation : Saturate  UpperLimit=[180*ones(5,1); 1]  LowerLimit=[-180*ones(5,1); 0]
  Signal Specification3 : SignalSpecification  Dimensions=6  OutDataType=sfix(16)  OutScaling=2^0
  Terminator : Terminator
  zeros : Constant  Value=zeros(6,1)  OutDataTypeMode=double  OutDataType=sfix(16)  OutScaling=2^0  OutDataTypeStr=double
  Joystick : Outport  OutDataType=sfix(16)  OutScaling=2^0
  Buttons : Outport  Port=2  OutDataType=sfix(16)  OutScaling=2^0
  wires:
  Demux/2 -> Terminator/1
  Demux/1 -> Signal Specification3/1
  Mux/1 -> Demux/1
  zeros/1 -> Mux/2
  Overlay/1 -> Mux/1
  Labels/1 -> S-Function/3
  Saturation/1 -> S-Function/2
  S-Function/2 -> Buttons/1
  Surfaces/1 -> Saturation/1
  S-Function/1 -> Joystick/1
  Positions/1 -> S-Function/1
  Signal Specification3/1 -> S-Function/4
